simulink model "Offline_DataImport_AND_ECGAnalysis_AND_SCGAnalysis"  (R2020b)
settings: Solver=FixedStepDiscrete  StartTime=0.0  StopTime=param_sim_time  FixedStep=1/fs  MaxStep=1/fs  RelTol=1e-3
undefined symbols (not defined in the file): analyses, fdesignblkfcn, fs, gcbh, param_tot_samples
libraries: dspstat3 x1
(part 1 of 5)
settings Model: PacingRate=100  Creator=rcord  LastModifiedBy=Rafael
settings SolverCC: ZeroCrossControl=DisableAll
settings DataIOCC: ExternalInput=[t, signals.ecg.input, signals.scg.input_x, signals.scg.input_y, signals.scg.input_z]  LoadExternalInput=on  SignalLogging=off  DSMLogging=off  SaveTime=off  ReturnWorkspaceOutputs=off  TimeSaveName=t_preprocessing  OutputSaveName=out_preprocessing  LoggingIntervals=[-inf,inf]
settings SFSimCC: CustomCodeUndefinedFunction=UseInterfaceOnly

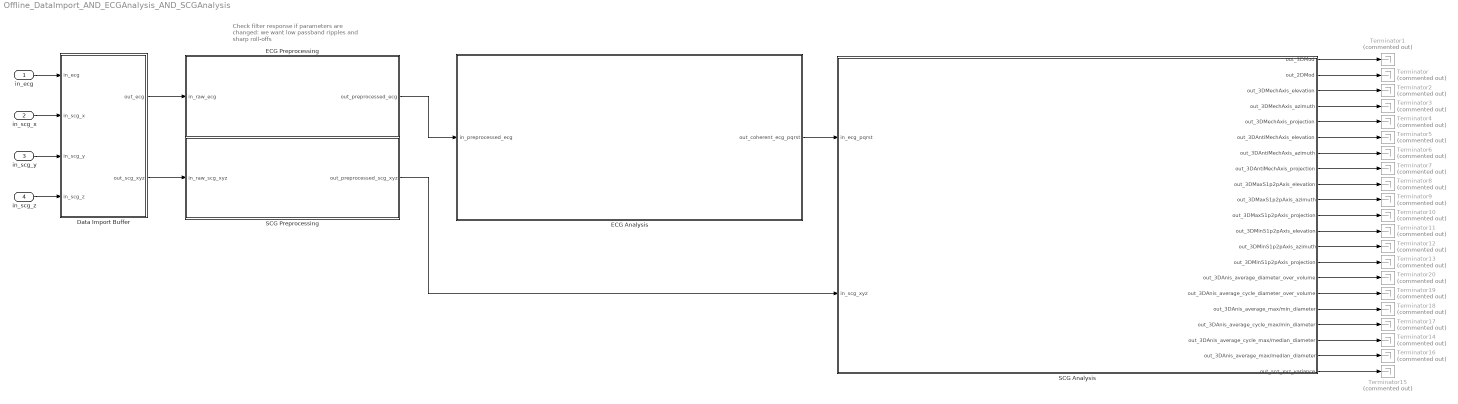
== system Offline_DataImport_AND_ECGAnalysis_AND_SCGAnalysis ==
  note: Check filter response if parameters are changed:
      | we want low passband ripples and sharp roll-offs
  in_ecg : Inport  SampleTime=1/fs
  in_scg_x : Inport  Port=2  SampleTime=1/fs
  in_scg_y : Inport  Port=3  SampleTime=1/fs
  in_scg_z : Inport  Port=4  SampleTime=1/fs
  Data Import Buffer : Subsystem
  ECG Analysis : Subsystem
      mask Display: image('C:\Users\Rafael\Dropbox\Post-Doc Research\ECG Analysis.jpg.png'); % Use "Edit Image" on toolstrip to change.
  ECG Preprocessing : Subsystem  mask{param_ecg_gain_mv=1000, param_ecg_fc_lo=2.05, param_ecg_fc_hi=36, param_ecg_trans_bw=2}
      mask prompts: param_ecg_gain_mv "mV Conversion Gain"; param_ecg_fc_lo "Low Passband Frequency Corner (Hz)"; param_ecg_fc_hi "High Passband Frequency Corner (Hz)"; param_ecg_trans_bw "Transition Bandwidth (Hz)"
      mask init:
      | assignin('base','param_ecg_gain_mv',param_ecg_gain_mv)
      | assignin('base','param_ecg_fc_lo',param_ecg_fc_lo)
      | assignin('base','param_ecg_fc_hi',param_ecg_fc_hi)
      | assignin('base','param_ecg_trans_bw',param_ecg_trans_bw)
      mask DialogControl DescGroupVar Prompt: ECG Preprocessing
      mask DialogControl DescTextVar Prompt: Preprocessing stage of the ECG. This involves conversion from V to mV and a filtfilt operation (i.e. a zero-phase FIR filtering) specified by the passband cornerns and transition bandwidth.
      mask Display: image('PreprocessingSymbol.jpg');
  SCG Analysis : Subsystem
      mask Display: image('C:\Users\Rafael\Dropbox\Post-Doc Research\SCG Analysis.png'); % Use "Edit Image" on toolstrip to change.
  SCG Preprocessing : Subsystem  mask{param_scg_gain_mg=3333, param_scg_fc_lo=7.5, param_scg_fc_hi=40, param_scg_trans_bw=2.5}
      mask prompts: param_scg_gain_mg "V to mg Conversion Gain"; param_scg_fc_lo "Low Passband Frequency Corner (Hz)"; param_scg_fc_hi "High Passband Frequency Corner (Hz)"; param_scg_trans_bw "Transition bandwidth"
      mask init:
      | assignin('base','param_scg_gain_mg',param_scg_gain_mg)
      | assignin('base','param_scg_fc_lo',param_scg_fc_lo)
      | assignin('base','param_scg_fc_hi',param_scg_fc_hi)
      | assignin('base','param_scg_trans_bw',param_scg_trans_bw)
      mask DialogControl DescGroupVar Prompt: SCG Preprocessing
      mask DialogControl DescTextVar Prompt: The SCG (x, y, and z) preprocessing block. This involves a V to mg conversion (determined by the transducer sensitivity) and a filtfilt operation. This filtfilt operation consists of a zero-phase FIR front-back filtering that is identical for each of the three cartesian acceleration components and is specified by the passband frequency corners and the transition bandwidth.
      mask Display: image('PreprocessingSymbol.jpg');
  Terminator{,1..20} (21 alike) : Terminator  Commented=on
  wires:
  in_ecg/1 -> Data Import Buffer/1(in_ecg)
  in_scg_x/1 -> Data Import Buffer/2(in_scg_x)
  in_scg_y/1 -> Data Import Buffer/3(in_scg_y)
  in_scg_z/1 -> Data Import Buffer/4(in_scg_z)
  Data Import Buffer/2(out_scg_xyz) -> SCG Preprocessing/1(in_raw_scg_xyz)
  Data Import Buffer/1(out_ecg) -> ECG Preprocessing/1(in_raw_ecg)
  ECG Preprocessing/1(out_preprocessed_ecg) -> ECG Analysis/1(in_preprocessed_ecg)
  SCG Preprocessing/1(out_preprocessed_scg_xyz) -> SCG Analysis/2(in_scg_xyz)
  ECG Analysis/1(out_coherent_ecg_pqrst) -> SCG Analysis/1(in_ecg_pqrst)
  SCG Analysis/1(out_3DMod) -> Terminator1/1
  SCG Analysis/2(out_2DMod) -> Terminator/1
  SCG Analysis/3(out_3DMechAxis_elevation) -> Terminator2/1
  SCG Analysis/4(out_3DMechAxis_azimuth) -> Terminator3/1
  SCG Analysis/5(out_3DMechAxis_projection) -> Terminator4/1
  SCG Analysis/6(out_3DAntiMechAxis_elevation) -> Terminator5/1
  SCG Analysis/7(out_3DAntiMechAxis_azimuth) -> Terminator6/1
  SCG Analysis/8(out_3DAntiMechAxis_projection) -> Terminator7/1
  SCG Analysis/9(out_3DMaxS1p2pAxis_elevation) -> Terminator8/1
  SCG Analysis/10(out_3DMaxS1p2pAxis_azimuth) -> Terminator9/1
  SCG Analysis/11(out_3DMaxS1p2pAxis_projection) -> Terminator10/1
  SCG Analysis/12(out_3DMinS1p2pAxis_elevation) -> Terminator11/1
  SCG Analysis/13(out_3DMinS1p2pAxis_azimuth) -> Terminator12/1
  SCG Analysis/14(out_3DMinS1p2pAxis_projection) -> Terminator13/1
  SCG Analysis/19(out_3DAnis_average_cycle_max/median_diameter) -> Terminator14/1
  SCG Analysis/21(out_scg_xyz_variance) -> Terminator15/1
  SCG Analysis/20(out_3DAnis_average_max/median_diameter) -> Terminator16/1
  SCG Analysis/18(out_3DAnis_average_cycle_max/min_diameter) -> Terminator17/1
  SCG Analysis/17(out_3DAnis_average_max/min_diameter) -> Terminator18/1
  SCG Analysis/16(out_3DAnis_average_cycle_diameter_over_volume) -> Terminator19/1
  SCG Analysis/15(out_3DAnis_average_diameter_over_volume) -> Terminator20/1

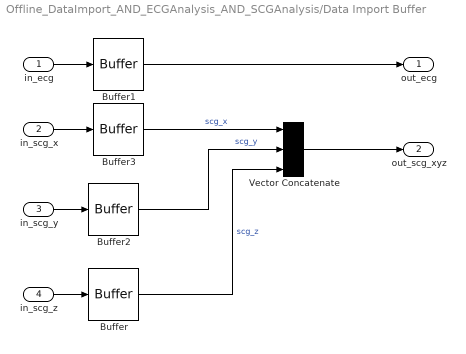
== system Offline_DataImport_AND_ECGAnalysis_AND_SCGAnalysis/Data Import Buffer ==
  in_ecg : Inport
  in_scg_x : Inport  Port=2
  in_scg_y : Inport  Port=3
  in_scg_z : Inport  Port=4
  Buffer{,1..3} (4 alike) : Buffer  N=param_tot_samples  OutputFrames=off
  Vector Concatenate : Concatenate  NumInputs=3  Mode=Multidimensional array  ConcatenateDimension=2
  out_ecg : Outport  VectorParamsAs1DForOutWhenUnconnected=off
  out_scg_xyz : Outport  Port=2  VectorParamsAs1DForOutWhenUnconnected=off
  wires:
  in_ecg/1 -> Buffer1/1
  Buffer/1 -> Vector Concatenate/3  "scg_z"
  Buffer3/1 -> Vector Concatenate/1  "scg_x"
  in_scg_x/1 -> Buffer3/1
  Vector Concatenate/1 -> out_scg_xyz/1
  Buffer1/1 -> out_ecg/1
  Buffer2/1 -> Vector Concatenate/2  "scg_y"
  in_scg_z/1 -> Buffer/1
  in_scg_y/1 -> Buffer2/1

== system Offline_DataImport_AND_ECGAnalysis_AND_SCGAnalysis/ECG Analysis ==
  in_preprocessed_ecg : Inport
  Enabled ECG Analysis Subsystem : Subsystem  TreatAsAtomicUnit=on
  out_coherent_ecg_pqrst : Outport
  wires:
  in_preprocessed_ecg/1 -> Enabled ECG Analysis Subsystem/Enable
  Enabled ECG Analysis Subsystem/1(coherent_ecg_pqrst) -> out_coherent_ecg_pqrst/1

== system Offline_DataImport_AND_ECGAnalysis_AND_SCGAnalysis/ECG Preprocessing ==
  in_raw_ecg : Inport
  Enabled ECG Preprocessing Subsystem : Subsystem  TreatAsAtomicUnit=on
  out_preprocessed_ecg : Outport  VectorParamsAs1DForOutWhenUnconnected=off
  wires:
  Enabled ECG Preprocessing Subsystem/1(Output) -> out_preprocessed_ecg/1
  in_raw_ecg/1 -> Enabled ECG Preprocessing Subsystem/Enable

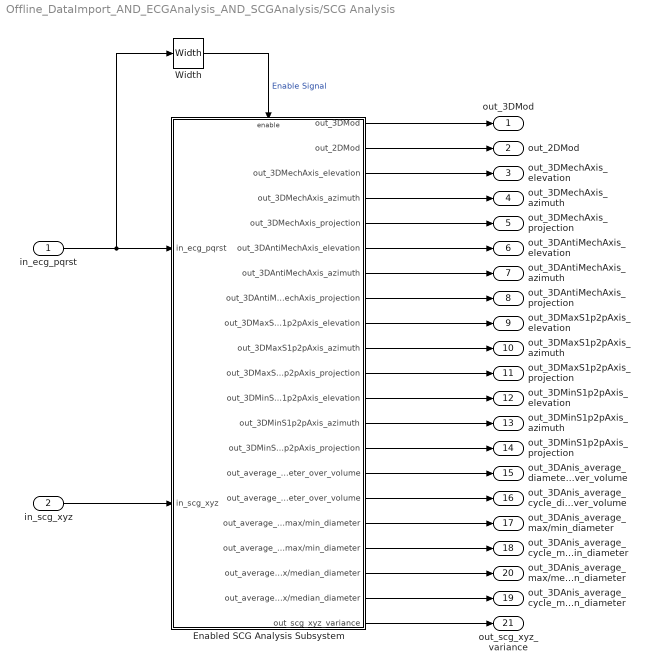
== system Offline_DataImport_AND_ECGAnalysis_AND_SCGAnalysis/SCG Analysis ==
  in_ecg_pqrst : Inport
  in_scg_xyz : Inport  Port=2
  Enabled SCG Analysis Subsystem : Subsystem  TreatAsAtomicUnit=on
  "Width " : Width
  out_3DMod : Outport  VectorParamsAs1DForOutWhenUnconnected=off
  out_2DMod : Outport  Port=2  VectorParamsAs1DForOutWhenUnconnected=off
  out_3DMechAxis_elevation : Outport  Port=3  VectorParamsAs1DForOutWhenUnconnected=off
  out_3DMechAxis_azimuth : Outport  Port=4  VectorParamsAs1DForOutWhenUnconnected=off
  out_3DMechAxis_projection : Outport  Port=5  VectorParamsAs1DForOutWhenUnconnected=off
  out_3DAntiMechAxis_elevation : Outport  Port=6  VectorParamsAs1DForOutWhenUnconnected=off
  out_3DAntiMechAxis_azimuth : Outport  Port=7  VectorParamsAs1DForOutWhenUnconnected=off
  out_3DAntiMechAxis_projection : Outport  Port=8  VectorParamsAs1DForOutWhenUnconnected=off
  out_3DMaxS1p2pAxis_elevation : Outport  Port=9  VectorParamsAs1DForOutWhenUnconnected=off
  out_3DMaxS1p2pAxis_azimuth : Outport  Port=10  VectorParamsAs1DForOutWhenUnconnected=off
  out_3DMaxS1p2pAxis_projection : Outport  Port=11  VectorParamsAs1DForOutWhenUnconnected=off
  out_3DMinS1p2pAxis_elevation : Outport  Port=12  VectorParamsAs1DForOutWhenUnconnected=off
  out_3DMinS1p2pAxis_azimuth : Outport  Port=13  VectorParamsAs1DForOutWhenUnconnected=off
  out_3DMinS1p2pAxis_projection : Outport  Port=14  VectorParamsAs1DForOutWhenUnconnected=off
  out_3DAnis_average_diameter_over_volume : Outport  Port=15  VectorParamsAs1DForOutWhenUnconnected=off
  out_3DAnis_average_cycle_diameter_over_volume : Outport  Port=16  VectorParamsAs1DForOutWhenUnconnected=off
  out_3DAnis_average_max/min_diameter : Outport  Port=17  VectorParamsAs1DForOutWhenUnconnected=off
  out_3DAnis_average_cycle_max/min_diameter : Outport  Port=18  VectorParamsAs1DForOutWhenUnconnected=off
  out_3DAnis_average_cycle_max/median_diameter : Outport  Port=19  VectorParamsAs1DForOutWhenUnconnected=off
  out_3DAnis_average_max/median_diameter : Outport  Port=20  VectorParamsAs1DForOutWhenUnconnected=off
  out_scg_xyz_variance : Outport  Port=21  VectorParamsAs1DForOutWhenUnconnected=off
  wires:
  Enabled SCG Analysis Subsystem/1(out_3DMod) -> out_3DMod/1
  Enabled SCG Analysis Subsystem/2(out_2DMod) -> out_2DMod/1
  in_scg_xyz/1 -> Enabled SCG Analysis Subsystem/2(in_scg_xyz)
  in_ecg_pqrst/1 -> "Width "/1, Enabled SCG Analysis Subsystem/1(in_ecg_pqrst)
  "Width "/1 -> Enabled SCG Analysis Subsystem/Enable  "Enable Signal"
  Enabled SCG Analysis Subsystem/3(out_3DMechAxis_elevation) -> out_3DMechAxis_elevation/1
  Enabled SCG Analysis Subsystem/4(out_3DMechAxis_azimuth) -> out_3DMechAxis_azimuth/1
  Enabled SCG Analysis Subsystem/14(out_3DMinS1p2pAxis_projection) -> out_3DMinS1p2pAxis_projection/1
  Enabled SCG Analysis Subsystem/13(out_3DMinS1p2pAxis_azimuth) -> out_3DMinS1p2pAxis_azimuth/1
  Enabled SCG Analysis Subsystem/12(out_3DMinS1p2pAxis_elevation) -> out_3DMinS1p2pAxis_elevation/1
  Enabled SCG Analysis Subsystem/11(out_3DMaxS1p2pAxis_projection) -> out_3DMaxS1p2pAxis_projection/1
  Enabled SCG Analysis Subsystem/10(out_3DMaxS1p2pAxis_azimuth) -> out_3DMaxS1p2pAxis_azimuth/1
  Enabled SCG Analysis Subsystem/9(out_3DMaxS1p2pAxis_elevation) -> out_3DMaxS1p2pAxis_elevation/1
  Enabled SCG Analysis Subsystem/8(out_3DAntiMechAxis_projection) -> out_3DAntiMechAxis_projection/1
  Enabled SCG Analysis Subsystem/7(out_3DAntiMechAxis_azimuth) -> out_3DAntiMechAxis_azimuth/1
  Enabled SCG Analysis Subsystem/6(out_3DAntiMechAxis_elevation) -> out_3DAntiMechAxis_elevation/1
  Enabled SCG Analysis Subsystem/5(out_3DMechAxis_projection) -> out_3DMechAxis_projection/1
  Enabled SCG Analysis Subsystem/20(out_average_cycle_cycle_max/median_diameter) -> out_3DAnis_average_cycle_max/median_diameter/1
  Enabled SCG Analysis Subsystem/15(out_average_diameter_over_volume) -> out_3DAnis_average_diameter_over_volume/1
  Enabled SCG Analysis Subsystem/21(out_scg_xyz_variance) -> out_scg_xyz_variance/1
  Enabled SCG Analysis Subsystem/16(out_average_cycle_diameter_over_volume) -> out_3DAnis_average_cycle_diameter_over_volume/1
  Enabled SCG Analysis Subsystem/17(out_average_max/min_diameter) -> out_3DAnis_average_max/min_diameter/1
  Enabled SCG Analysis Subsystem/18(out_average_cycle_max/min_diameter) -> out_3DAnis_average_cycle_max/min_diameter/1
  Enabled SCG Analysis Subsystem/19(out_average_max/median_diameter) -> out_3DAnis_average_max/median_diameter/1

== system Offline_DataImport_AND_ECGAnalysis_AND_SCGAnalysis/SCG Preprocessing ==
  in_raw_scg_xyz : Inport
  Enabled SCG Preprocessing Subsystem : Subsystem  TreatAsAtomicUnit=on
  out_preprocessed_scg_xyz : Outport  VectorParamsAs1DForOutWhenUnconnected=off
  wires:
  Enabled SCG Preprocessing Subsystem/1(out_preprocessed_scg_xyz) -> out_preprocessed_scg_xyz/1
  in_raw_scg_xyz/1 -> Enabled SCG Preprocessing Subsystem/Enable

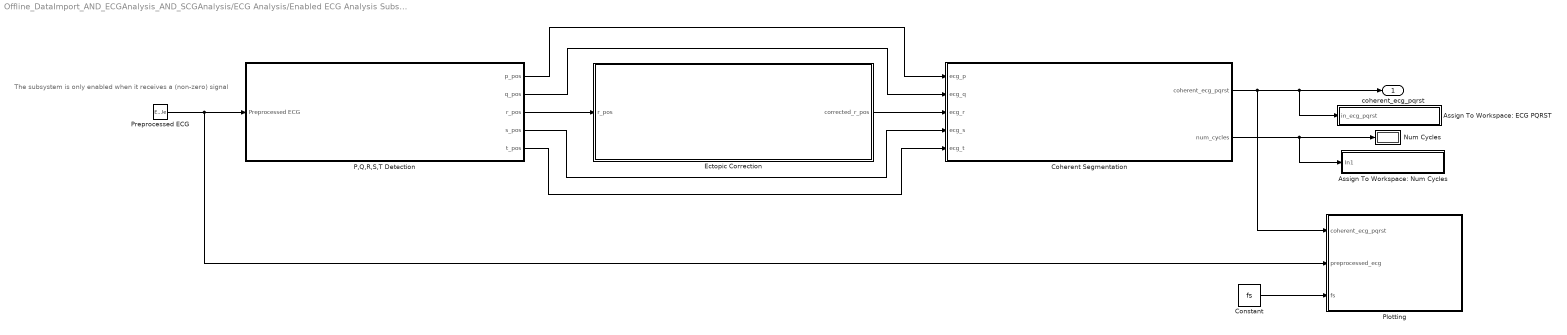
== system Offline_DataImport_AND_ECGAnalysis_AND_SCGAnalysis/ECG Analysis/Enabled ECG Analysis Subsystem ==
  note: The subsystem is only enabled when it receives a (non-zero) signal
  Preprocessed ECG : EnablePort  PropagateVarSize=During execution  ShowOutputPort=on
  Assign To Workspace: ECG PQRST : Subsystem
      mask Display: disp('Assign: out_ecg_pqrst')
  Assign To Workspace: Num Cycles : Subsystem
      mask Display: disp('Assign: out_ecg_num_cycles')
  Coherent Segmentation : Subsystem
      mask Display: image('C:\Users\Rafael\Dropbox\Post-Doc Research\Coherent ECG.jpg'); % Use "Edit Image" on toolstrip to change.
  Constant : Constant  Value=fs
  Ectopic Correction : Subsystem  mask{max_hr=200, max_rr_dev=40}
      mask prompts: max_hr "Maximum Heart Rate (in bpm)"; max_rr_dev "Maximum RR Deviation (in bpm)"
      mask DialogControl DescGroupVar Prompt: Ectopic Correction
      mask DialogControl DescTextVar Prompt: Specify the ectopic detection parameters. What will be defined as an ectopic cycle and removed from further analysis? Maximum heart rate specifies the upper limit of heart rate - any cycles with RR intervals corresponding to heart rates above this limit will be considered ectopic. Maximum RR deviation - any cycles with RR intervals greater or less than this deviation from the average RR will be considered ectopic.
      mask Display: image('C:\Users\Rafael\Dropbox\Post-Doc Research\Tachogram.jpg'); % Use "Edit Image" on toolstrip to change.
  Num Cycles : Display
  P,Q,R,S,T Detection : Subsystem  mask{ecg_algo=PQRST waves - Multi-level Teager Energy Operator}
      mask prompts: ecg_algo "Choose one:"
      mask init:
      | if ecg_algo == 1
      |     param_ecg_algo = 'Pan-Tompkins';
      | elseif ecg_algo == 2
      |     param_ecg_algo = 'Phase Space';
      | elseif ecg_algo == 3
      |     param_ecg_algo = 'Filter Bank';
      | elseif ecg_algo == 4
      |     param_ecg_algo = 'State Machine';
      | elseif ecg_algo == 5
      |     param_ecg_algo = 'Multi-level Teager Energy Operator';
      | end
      | 
      | assignin('base','param_ecg_algo', param_ecg_algo)
      mask TypeOptions ecg_algo: R wave  - Pan-Tompkins | R wave - Phase space | R wave - Filter bank | QRST waves - State machine | PQRST waves - Multi-level Teager Energy Operator
      mask DialogControl DescGroupVar Prompt: ECG PQRST Detection
      mask DialogControl DescTextVar Prompt: Select detected waveform(s) and corresponding detection aglorithm.
      mask DialogControl ParameterGroupVar Prompt: Desired wave(s) and Algorithm
      mask Display: image('C:\Users\Rafael\Dropbox\Post-Doc Research\Labelled ECG.jpg'); % Use "Edit Image" on toolstrip to change.
  Plotting : MATLAB Function  TreatAsAtomicUnit=on
  coherent_ecg_pqrst : Outport
  wires:
  Preprocessed ECG/1 -> P,Q,R,S,T Detection/1(Preprocessed ECG), Plotting/2(preprocessed_ecg)
  P,Q,R,S,T Detection/3(r_pos) -> Ectopic Correction/1(r_pos)
  Constant/1 -> Plotting/3(fs)
  Coherent Segmentation/2(num_cycles) -> Assign To Workspace: Num Cycles/1(In1), Num Cycles/1
  Ectopic Correction/1(corrected_r_pos) -> Coherent Segmentation/3(ecg_r)
  Coherent Segmentation/1(coherent_ecg_pqrst) -> Assign To Workspace: ECG PQRST/1(in_ecg_pqrst), coherent_ecg_pqrst/1, Plotting/1(coherent_ecg_pqrst)
  P,Q,R,S,T Detection/5(t_pos) -> Coherent Segmentation/5(ecg_t)
  P,Q,R,S,T Detection/4(s_pos) -> Coherent Segmentation/4(ecg_s)
  P,Q,R,S,T Detection/1(p_pos) -> Coherent Segmentation/1(ecg_p)
  P,Q,R,S,T Detection/2(q_pos) -> Coherent Segmentation/2(ecg_q)

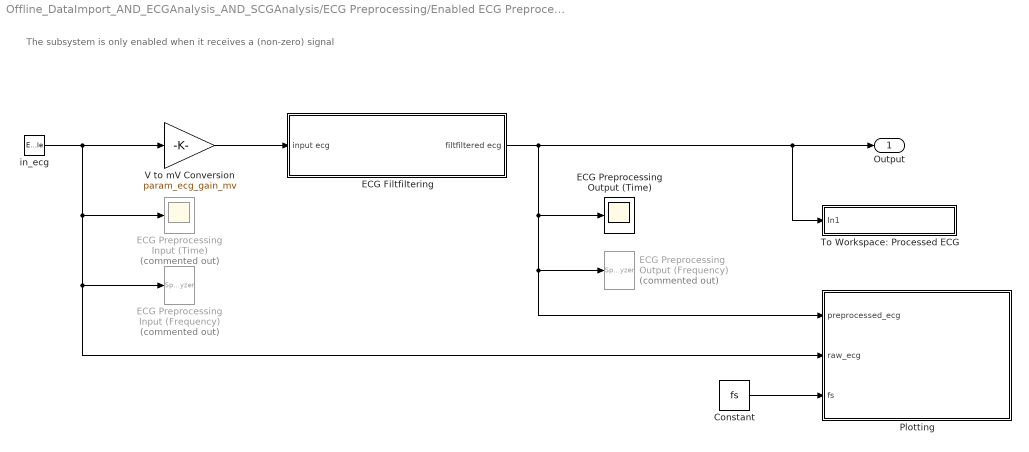
== system Offline_DataImport_AND_ECGAnalysis_AND_SCGAnalysis/ECG Preprocessing/Enabled ECG Preprocessing Subsystem ==
  note: The subsystem is only enabled when it receives a (non-zero) signal
  in_ecg : EnablePort  ShowOutputPort=on
  Constant : Constant  Value=fs
  ECG Filtfiltering : Subsystem
  ECG Preprocessing Input (Frequency) : SpectrumAnalyzer  Commented=on
  ECG Preprocessing Input (Time) : Scope  Commented=on
  ECG Preprocessing Output (Frequency) : SpectrumAnalyzer  Commented=on
  ECG Preprocessing Output (Time) : Scope
  Plotting : MATLAB Function  TreatAsAtomicUnit=on
  To Workspace: Processed ECG : Subsystem
      mask Display: disp('out_ecg_preprocessing')
  V to mV Conversion : Gain  Gain=param_ecg_gain_mv
  Output : Outport  VectorParamsAs1DForOutWhenUnconnected=off
  wires:
  V to mV Conversion/1 -> ECG Filtfiltering/1(input ecg)
  in_ecg/1 -> V to mV Conversion/1, ECG Preprocessing Input (Time)/1, Plotting/2(raw_ecg), ECG Preprocessing Input (Frequency)/1
  ECG Filtfiltering/1(filtfiltered ecg) -> To Workspace: Processed ECG/1(In1), Output/1, ECG Preprocessing Output (Time)/1, Plotting/1(preprocessed_ecg), ECG Preprocessing Output (Frequency)/1
  Constant/1 -> Plotting/3(fs)

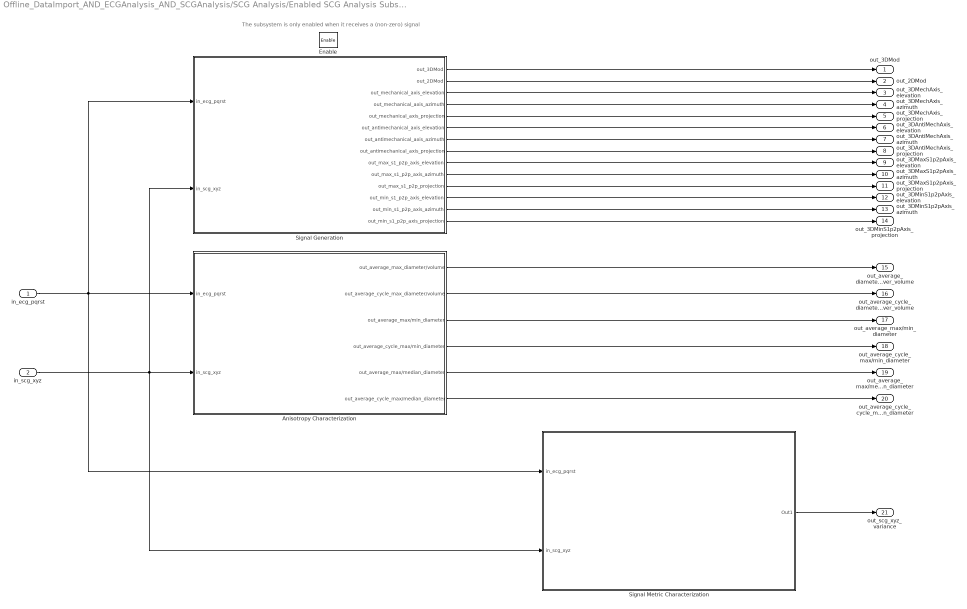
== system Offline_DataImport_AND_ECGAnalysis_AND_SCGAnalysis/SCG Analysis/Enabled SCG Analysis Subsystem ==
  note: The subsystem is only enabled when it receives a (non-zero) signal
  in_ecg_pqrst : Inport
  in_scg_xyz : Inport  Port=2
  Enable : EnablePort  StatesWhenEnabling=reset  PropagateVarSize=During execution
  Anisotropy Characterization : Subsystem
      mask Display: image('C:\Users\Rafael\Dropbox\Post-Doc Research\Anisotropy.png'); % Use "Edit Image" on toolstrip to change.
  Signal Generation : Subsystem
      mask Display: image('C:\Users\Rafael\Dropbox\Post-Doc Research\Signal Generation.png'); % Use "Edit Image" on toolstrip to change.
  Signal Metric Characterization : Subsystem
      mask Display: image('C:\Users\Rafael\Dropbox\Post-Doc Research\SCGAnalysisSymbol.jpg'); % Use "Edit Image" on toolstrip to change.
  out_3DMod : Outport  VectorParamsAs1DForOutWhenUnconnected=off
  out_2DMod : Outport  Port=2  VectorParamsAs1DForOutWhenUnconnected=off
  out_3DMechAxis_elevation : Outport  Port=3  VectorParamsAs1DForOutWhenUnconnected=off
  out_3DMechAxis_azimuth : Outport  Port=4  VectorParamsAs1DForOutWhenUnconnected=off
  out_3DMechAxis_projection : Outport  Port=5  VectorParamsAs1DForOutWhenUnconnected=off
  out_3DAntiMechAxis_elevation : Outport  Port=6  VectorParamsAs1DForOutWhenUnconnected=off
  out_3DAntiMechAxis_azimuth : Outport  Port=7  VectorParamsAs1DForOutWhenUnconnected=off
  out_3DAntiMechAxis_projection : Outport  Port=8  VectorParamsAs1DForOutWhenUnconnected=off
  out_3DMaxS1p2pAxis_elevation : Outport  Port=9  VectorParamsAs1DForOutWhenUnconnected=off
  out_3DMaxS1p2pAxis_azimuth : Outport  Port=10  VectorParamsAs1DForOutWhenUnconnected=off
  out_3DMaxS1p2pAxis_projection : Outport  Port=11  VectorParamsAs1DForOutWhenUnconnected=off
  out_3DMinS1p2pAxis_elevation : Outport  Port=12  VectorParamsAs1DForOutWhenUnconnected=off
  out_3DMinS1p2pAxis_azimuth : Outport  Port=13  VectorParamsAs1DForOutWhenUnconnected=off
  out_3DMinS1p2pAxis_projection : Outport  Port=14  VectorParamsAs1DForOutWhenUnconnected=off
  out_average_diameter_over_volume : Outport  Port=15  VectorParamsAs1DForOutWhenUnconnected=off
  out_average_cycle_diameter_over_volume : Outport  Port=16  VectorParamsAs1DForOutWhenUnconnected=off
  out_average_max/min_diameter : Outport  Port=17  VectorParamsAs1DForOutWhenUnconnected=off
  out_average_cycle_max/min_diameter : Outport  Port=18  VectorParamsAs1DForOutWhenUnconnected=off
  out_average_max/median_diameter : Outport  Port=19  VectorParamsAs1DForOutWhenUnconnected=off
  out_average_cycle_cycle_max/median_diameter : Outport  Port=20  VectorParamsAs1DForOutWhenUnconnected=off
  out_scg_xyz_variance : Outport  Port=21  VectorParamsAs1DForOutWhenUnconnected=off
  wires:
  Signal Generation/2(out_2DMod) -> out_2DMod/1
  Signal Generation/1(out_3DMod) -> out_3DMod/1
  in_scg_xyz/1 -> Signal Generation/2(in_scg_xyz), Signal Metric Characterization/2(in_scg_xyz), Anisotropy Characterization/2(in_scg_xyz)
  in_ecg_pqrst/1 -> Anisotropy Characterization/1(in_ecg_pqrst), Signal Generation/1(in_ecg_pqrst), Signal Metric Characterization/1(in_ecg_pqrst)
  Signal Generation/3(out_mechanical_axis_elevation) -> out_3DMechAxis_elevation/1
  Signal Generation/4(out_mechanical_axis_azimuth) -> out_3DMechAxis_azimuth/1
  Signal Generation/5(out_mechanical_axis_projection) -> out_3DMechAxis_projection/1
  Signal Generation/6(out_antimechanical_axis_elevation) -> out_3DAntiMechAxis_elevation/1
  Signal Generation/7(out_antimechanical_axis_azimuth) -> out_3DAntiMechAxis_azimuth/1
  Signal Generation/8(out_antimechanical_axis_projection) -> out_3DAntiMechAxis_projection/1
  Signal Generation/9(out_max_s1_p2p_axis_elevation) -> out_3DMaxS1p2pAxis_elevation/1
  Signal Generation/10(out_max_s1_p2p_axis_azimuth) -> out_3DMaxS1p2pAxis_azimuth/1
  Signal Generation/11(out_max_s1_p2p_projection) -> out_3DMaxS1p2pAxis_projection/1
  Signal Generation/12(out_min_s1_p2p_axis_elevation) -> out_3DMinS1p2pAxis_elevation/1
  Signal Generation/13(out_min_s1_p2p_axis_azimuth) -> out_3DMinS1p2pAxis_azimuth/1
  Signal Generation/14(out_min_s1_p2p_axis_projection) -> out_3DMinS1p2pAxis_projection/1
  Anisotropy Characterization/1(out_average_max_diameter/volume) -> out_average_diameter_over_volume/1
  Signal Metric Characterization/1(Out1) -> out_scg_xyz_variance/1
  Anisotropy Characterization/2(out_average_cycle_max_diameter/volume) -> out_average_cycle_diameter_over_volume/1
  Anisotropy Characterization/3(out_average_max/min_diameter) -> out_average_max/min_diameter/1
  Anisotropy Characterization/4(out_average_cycle_max/min_diameter) -> out_average_cycle_max/min_diameter/1
  Anisotropy Characterization/5(out_average_max/median_diameter) -> out_average_max/median_diameter/1
  Anisotropy Characterization/6(out_average_cycle_max/median_diameter) -> out_average_cycle_cycle_max/median_diameter/1

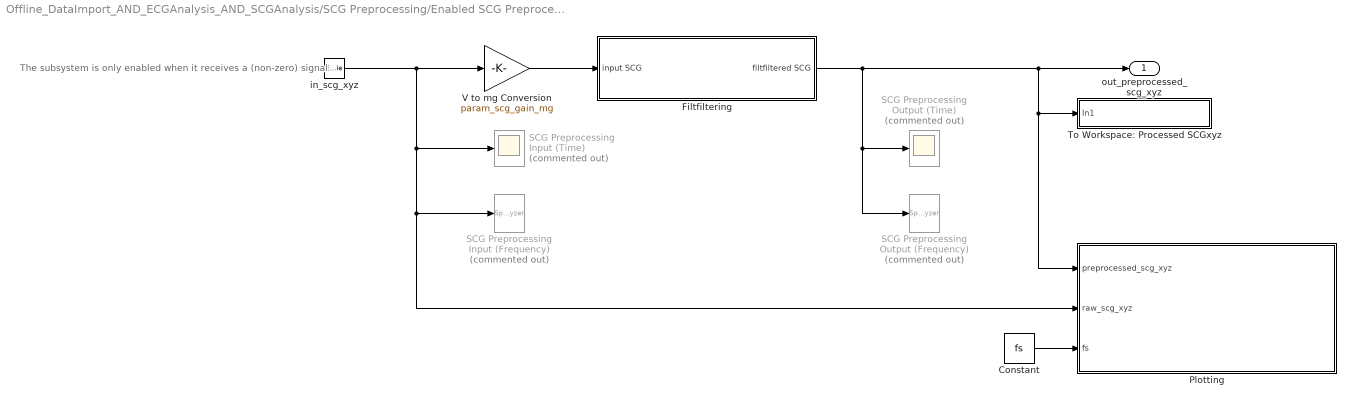
== system Offline_DataImport_AND_ECGAnalysis_AND_SCGAnalysis/SCG Preprocessing/Enabled SCG Preprocessing Subsystem ==
  note: The subsystem is only enabled when it receives a (non-zero) signal
  in_scg_xyz : EnablePort  ShowOutputPort=on
  Constant : Constant  Value=fs
  Filtfiltering : Subsystem
  Plotting : MATLAB Function  TreatAsAtomicUnit=on
  SCG Preprocessing Input (Frequency) : SpectrumAnalyzer  Commented=on
  SCG Preprocessing Input (Time) : Scope  Commented=on
  SCG Preprocessing Output (Frequency) : SpectrumAnalyzer  Commented=on
  SCG Preprocessing Output (Time) : Scope  Commented=on
  To Workspace: Processed SCGxyz : Subsystem
      mask Display: disp('out_scg_xyz_preprocessing')
  V to mg Conversion : Gain  Gain=param_scg_gain_mg
  out_preprocessed_scg_xyz : Outport  VectorParamsAs1DForOutWhenUnconnected=off
  wires:
  V to mg Conversion/1 -> Filtfiltering/1(" input SCG")
  Filtfiltering/1(filtfiltered SCG) -> out_preprocessed_scg_xyz/1, To Workspace: Processed SCGxyz/1(In1), Plotting/1(preprocessed_scg_xyz), SCG Preprocessing Output (Frequency)/1, SCG Preprocessing Output (Time)/1
  Constant/1 -> Plotting/3(fs)
  in_scg_xyz/1 -> V to mg Conversion/1, Plotting/2(raw_scg_xyz), SCG Preprocessing Input (Frequency)/1, SCG Preprocessing Input (Time)/1

== system Offline_DataImport_AND_ECGAnalysis_AND_SCGAnalysis/ECG Analysis/Enabled ECG Analysis Subsystem/Assign To Workspace: ECG PQRST ==
  in_ecg_pqrst : Inport
  Enable Selector : Selector  NumberOfDimensions=2  InputPortWidth=3  IndexOptions=Index vector (dialog),Index vector (dialog)  Indices=[1],[3]  OutputSizes=1,1
  Enabled To Workspace ECG PQRST : Subsystem  TreatAsAtomicUnit=on
  wires:
  in_ecg_pqrst/1 -> Enable Selector/1, Enabled To Workspace ECG PQRST/1(in_ecg_pqrst)
  Enable Selector/1 -> Enabled To Workspace ECG PQRST/Enable  "Enable"

== system Offline_DataImport_AND_ECGAnalysis_AND_SCGAnalysis/ECG Analysis/Enabled ECG Analysis Subsystem/Assign To Workspace: Num Cycles ==
  In1 : Inport
  Enabled To Workspace ECG Num Cycles : Subsystem  TreatAsAtomicUnit=on
  wires:
  In1/1 -> Enabled To Workspace ECG Num Cycles/Enable

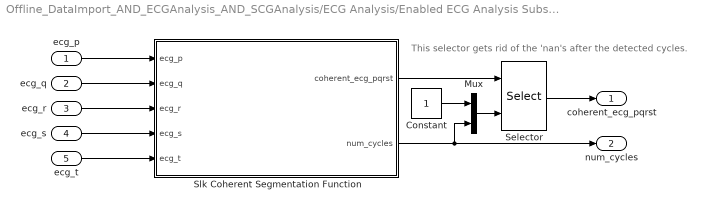
== system Offline_DataImport_AND_ECGAnalysis_AND_SCGAnalysis/ECG Analysis/Enabled ECG Analysis Subsystem/Coherent Segmentation ==
  note: This selector gets rid of the 'nan's after the detected cycles.
  ecg_p : Inport
  ecg_q : Inport  Port=2
  ecg_r : Inport  Port=3
  ecg_s : Inport  Port=4
  ecg_t : Inport  Port=5
  Constant : Constant
  Mux : Mux  Inputs=2
  Selector : Selector  NumberOfDimensions=2  InputPortWidth=3  IndexOptions=Starting and ending indices (port),Index vector (dialog)  Indices=[1 3],[1 2 3 3 5]  OutputSizes=1,1
  Slk Coherent Segmentation Function : MATLAB Function  TreatAsAtomicUnit=on
  coherent_ecg_pqrst : Outport
  num_cycles : Outport  Port=2
  wires:
  ecg_q/1 -> Slk Coherent Segmentation Function/2(ecg_q)
  ecg_s/1 -> Slk Coherent Segmentation Function/4(ecg_s)
  ecg_p/1 -> Slk Coherent Segmentation Function/1(ecg_p)
  ecg_r/1 -> Slk Coherent Segmentation Function/3(ecg_r)
  ecg_t/1 -> Slk Coherent Segmentation Function/5(ecg_t)
  Constant/1 -> Mux/1
  Mux/1 -> Selector/2
  Slk Coherent Segmentation Function/1(coherent_ecg_pqrst) -> Selector/1
  Selector/1 -> coherent_ecg_pqrst/1
  Slk Coherent Segmentation Function/2(num_cycles) -> num_cycles/1, Mux/2

== system Offline_DataImport_AND_ECGAnalysis_AND_SCGAnalysis/ECG Analysis/Enabled ECG Analysis Subsystem/Ectopic Correction ==
  r_pos : Inport
  Constant : Constant  Value=max_hr
  Constant1 : Constant  Value=max_rr_dev
  Constant2 : Constant  Value=fs
  Ectopic Correction : MATLAB Function  TreatAsAtomicUnit=on
  corrected_r_pos : Outport
  wires:
  Ectopic Correction/1(corrected_r_pos) -> corrected_r_pos/1
  Constant2/1 -> Ectopic Correction/1(fs)
  Constant/1 -> Ectopic Correction/2(max_hr)
  Constant1/1 -> Ectopic Correction/3(max_rr_dev)
  r_pos/1 -> Ectopic Correction/4(r_pos)

== system Offline_DataImport_AND_ECGAnalysis_AND_SCGAnalysis/ECG Analysis/Enabled ECG Analysis Subsystem/P,Q,R,S,T Detection ==
  Preprocessed ECG : Inport
  Constant : Constant  Value=fs
  Constant1 : Constant  Value=ecg_algo
  Wrapped BioSigKit ECG PQRST Detection : MATLAB Function  TreatAsAtomicUnit=on
  p_pos : Outport
      settings: VarSizeSig=Yes
  q_pos : Outport  Port=2
      settings: VarSizeSig=Yes
  r_pos : Outport  Port=3
      settings: VarSizeSig=Yes
  s_pos : Outport  Port=4
      settings: VarSizeSig=Yes
  t_pos : Outport  Port=5
      settings: VarSizeSig=Yes
  wires:
  Preprocessed ECG/1 -> Wrapped BioSigKit ECG PQRST Detection/2(preprocessed_ecg)
  Constant/1 -> Wrapped BioSigKit ECG PQRST Detection/1(fs)
  Wrapped BioSigKit ECG PQRST Detection/1(ecg_p) -> p_pos/1
  Wrapped BioSigKit ECG PQRST Detection/2(ecg_q) -> q_pos/1
  Wrapped BioSigKit ECG PQRST Detection/3(ecg_r) -> r_pos/1
  Wrapped BioSigKit ECG PQRST Detection/4(ecg_s) -> s_pos/1
  Wrapped BioSigKit ECG PQRST Detection/5(ecg_t) -> t_pos/1
  Constant1/1 -> Wrapped BioSigKit ECG PQRST Detection/3(ecg_algo)

== system Offline_DataImport_AND_ECGAnalysis_AND_SCGAnalysis/ECG Preprocessing/Enabled ECG Preprocessing Subsystem/ECG Filtfiltering ==
  input ecg : Inport
  Bandpass Filter 1 : Subsystem  DialogController=fdesignblkfcn  InitFcn=fdesignblkfcn(gcbh, {'InitFcn'});  mask(Bandpass Filter){}
      mask help: Design a bandpass filter
      settings: CopyFcn=fdesignblkfcn(gcbh, {'CopyFcn'});
      mask Help: helpview(mapfilelocation('dsp'), 'dspbandpassfilter');
      mask Display: disp('Bandpass');
  Bandpass Filter 2 : Subsystem  DialogController=fdesignblkfcn  InitFcn=fdesignblkfcn(gcbh, {'InitFcn'});  mask(Bandpass Filter){}
      mask help: Design a bandpass filter
      settings: CopyFcn=fdesignblkfcn(gcbh, {'CopyFcn'});
      mask Help: helpview(mapfilelocation('dsp'), 'dspbandpassfilter');
      mask Display: disp('Bandpass');
  Flip : DSPFlip
  Flip1 : DSPFlip
  filtfiltered ecg : Outport  VectorParamsAs1DForOutWhenUnconnected=off
  wires:
  Flip/1 -> Bandpass Filter 2/1(In)
  input ecg/1 -> Bandpass Filter 1/1(In)
  Flip1/1 -> filtfiltered ecg/1
  Bandpass Filter 1/1(Out) -> Flip/1
  Bandpass Filter 2/1(Out) -> Flip1/1

== system Offline_DataImport_AND_ECGAnalysis_AND_SCGAnalysis/ECG Preprocessing/Enabled ECG Preprocessing Subsystem/To Workspace: Processed ECG ==
  In1 : Inport
  Enabled To Workspace ECG Subsystem : Subsystem  TreatAsAtomicUnit=on
  wires:
  In1/1 -> Enabled To Workspace ECG Subsystem/Enable, Enabled To Workspace ECG Subsystem/1(In1)

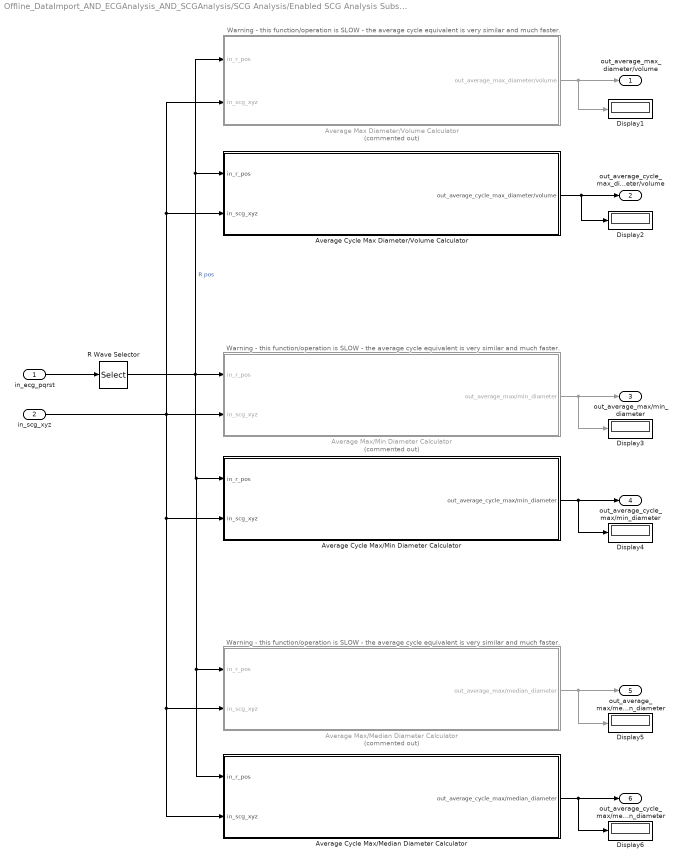
== system Offline_DataImport_AND_ECGAnalysis_AND_SCGAnalysis/SCG Analysis/Enabled SCG Analysis Subsystem/Anisotropy Characterization ==
  note: Warning - this function/operation is SLOW - the average cycle equivalent is very similar and much faster.
  note: Warning - this function/operation is SLOW - the average cycle equivalent is very similar and much faster.
  note: Warning - this function/operation is SLOW - the average cycle equivalent is very similar and much faster.
  in_ecg_pqrst : Inport
  in_scg_xyz : Inport  Port=2
  Average Cycle Max Diameter/Volume Calculator : Subsystem
  Average Cycle Max/Median Diameter Calculator : Subsystem
  Average Cycle Max/Min Diameter Calculator : Subsystem
  Average Max Diameter/Volume Calculator : Subsystem  Commented=on
  Average Max/Median Diameter Calculator : Subsystem  Commented=on
  Average Max/Min Diameter Calculator : Subsystem  Commented=on
  Display{1..6} (6 alike) : Display
  R Wave Selector : Selector  NumberOfDimensions=2  InputPortWidth=3  IndexOptions=Select all,Index vector (dialog)  Indices=[1 3],3  OutputSizes=1,1
  out_average_max_diameter/volume : Outport
  out_average_cycle_max_diameter/volume : Outport  Port=2
  out_average_max/min_diameter : Outport  Port=3
  out_average_cycle_max/min_diameter : Outport  Port=4
  out_average_max/median_diameter : Outport  Port=5
  out_average_cycle_max/median_diameter : Outport  Port=6
  wires:
  Average Max Diameter/Volume Calculator/1(out_average_max_diameter/volume) -> out_average_max_diameter/volume/1, Display1/1
  in_ecg_pqrst/1 -> R Wave Selector/1
  in_scg_xyz/1 -> Average Max Diameter/Volume Calculator/2(in_scg_xyz), Average Cycle Max Diameter/Volume Calculator/2(in_scg_xyz), Average Cycle Max/Median Diameter Calculator/2(in_scg_xyz), Average Max/Median Diameter Calculator/2(in_scg_xyz), Average Cycle Max/Min Diameter Calculator/2(in_scg_xyz), Average Max/Min Diameter Calculator/2(in_scg_xyz)
  Average Cycle Max Diameter/Volume Calculator/1(out_average_cycle_max_diameter/volume) -> Display2/1, out_average_cycle_max_diameter/volume/1
  R Wave Selector/1 -> Average Cycle Max Diameter/Volume Calculator/1(in_r_pos), Average Max Diameter/Volume Calculator/1(in_r_pos), Average Max/Min Diameter Calculator/1(in_r_pos), Average Cycle Max/Median Diameter Calculator/1(in_r_pos), Average Max/Median Diameter Calculator/1(in_r_pos), Average Cycle Max/Min Diameter Calculator/1(in_r_pos)  "R pos"
  Average Max/Min Diameter Calculator/1(out_average_max/min_diameter) -> out_average_max/min_diameter/1, Display3/1
  Average Cycle Max/Min Diameter Calculator/1(out_average_cycle_max/min_diameter) -> Display4/1, out_average_cycle_max/min_diameter/1
  Average Max/Median Diameter Calculator/1(out_average_max/median_diameter) -> Display5/1, out_average_max/median_diameter/1
  Average Cycle Max/Median Diameter Calculator/1(out_average_cycle_max/median_diameter) -> out_average_cycle_max/median_diameter/1, Display6/1

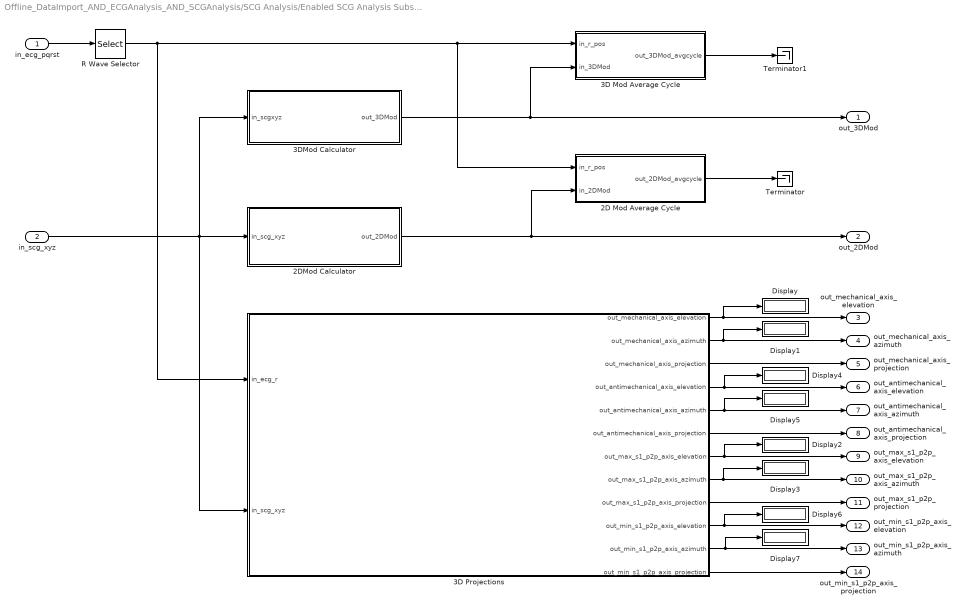
== system Offline_DataImport_AND_ECGAnalysis_AND_SCGAnalysis/SCG Analysis/Enabled SCG Analysis Subsystem/Signal Generation ==
  in_ecg_pqrst : Inport
  in_scg_xyz : Inport  Port=2
  2D Mod Average Cycle : Subsystem
  2DMod Calculator : Subsystem  mask{xyz2Dcombo=xz (transverse plane)}
      mask prompts: xyz2Dcombo "2D component combination:"
      mask init:
      | if xyz2Dcombo == 1
      |     param_2Dxyzcombo = 'xy';
      | elseif xyz2Dcombo == 2
      |     param_2Dxyzcombo = 'yz';
      | elseif xyz2Dcombo == 3
      |     param_2Dxyzcombo = 'xz';
      | end
      | 
      | assignin('base','param_2Dxyzcombo', param_2Dxyzcombo)
      mask TypeOptions xyz2Dcombo: xy (coronal plane) | yz (sagittal plane) | xz (transverse plane)
      mask DialogControl DescGroupVar Prompt: 2D Modulus Calculator
      mask DialogControl DescTextVar Prompt: Subsystem to calculate a 2D modulus signal from a user-specified combination of any two of the SCG x, y, or z components.
  3D Mod Average Cycle : Subsystem
  3D Projections : Subsystem
      mask Display: image('C:\Users\Rafael\Dropbox\Post-Doc Research\Coordinate Frames with Signals.png'); % Use "Edit Image" on toolstrip to change.
  3DMod Calculator : Subsystem
  Display{,1..7} (8 alike) : Display
  R Wave Selector : Selector  NumberOfDimensions=2  InputPortWidth=3  IndexOptions=Select all,Index vector (dialog)  Indices=[1 3],3  OutputSizes=1,1
  Terminator : Terminator
  Terminator1 : Terminator
  out_3DMod : Outport
  out_2DMod : Outport  Port=2
  out_mechanical_axis_elevation : Outport  Port=3
  out_mechanical_axis_azimuth : Outport  Port=4
  out_mechanical_axis_projection : Outport  Port=5
  out_antimechanical_axis_elevation : Outport  Port=6
  out_antimechanical_axis_azimuth : Outport  Port=7
  out_antimechanical_axis_projection : Outport  Port=8
  out_max_s1_p2p_axis_elevation : Outport  Port=9
  out_max_s1_p2p_axis_azimuth : Outport  Port=10
  out_max_s1_p2p_projection : Outport  Port=11
  out_min_s1_p2p_axis_elevation : Outport  Port=12
  out_min_s1_p2p_axis_azimuth : Outport  Port=13
  out_min_s1_p2p_axis_projection : Outport  Port=14
  wires:
  3DMod Calculator/1(out_3DMod) -> out_3DMod/1, 3D Mod Average Cycle/2(in_3DMod)
  2DMod Calculator/1(out_2DMod) -> 2D Mod Average Cycle/2(in_2DMod), out_2DMod/1
  2D Mod Average Cycle/1(out_2DMod_avgcycle) -> Terminator/1
  3D Mod Average Cycle/1(out_3DMod_avgcycle) -> Terminator1/1
  R Wave Selector/1 -> 3D Mod Average Cycle/1(in_r_pos), 2D Mod Average Cycle/1(in_r_pos), 3D Projections/1(in_ecg_r)
  in_ecg_pqrst/1 -> R Wave Selector/1
  in_scg_xyz/1 -> 3DMod Calculator/1(in_scgxyz), 2DMod Calculator/1(in_scg_xyz), 3D Projections/2(in_scg_xyz)
  3D Projections/4(out_antimechanical_axis_elevation) -> out_antimechanical_axis_elevation/1, Display4/1
  3D Projections/2(out_mechanical_axis_azimuth) -> Display1/1, out_mechanical_axis_azimuth/1
  3D Projections/10(out_min_s1_p2p_axis_elevation) -> Display6/1, out_min_s1_p2p_axis_elevation/1
  3D Projections/5(out_antimechanical_axis_azimuth) -> out_antimechanical_axis_azimuth/1, Display5/1
  3D Projections/8(out_max_s1_p2p_axis_azimuth) -> Display3/1, out_max_s1_p2p_axis_azimuth/1
  3D Projections/6(out_antimechanical_axis_projection) -> out_antimechanical_axis_projection/1
  3D Projections/7(out_max_s1_p2p_axis_elevation) -> out_max_s1_p2p_axis_elevation/1, Display2/1
  3D Projections/11(out_min_s1_p2p_axis_azimuth) -> out_min_s1_p2p_axis_azimuth/1, Display7/1
  3D Projections/12(out_min_s1_p2p_axis_projection) -> out_min_s1_p2p_axis_projection/1
  3D Projections/9(out_max_s1_p2p_axis_projection) -> out_max_s1_p2p_projection/1
  3D Projections/1(out_mechanical_axis_elevation) -> Display/1, out_mechanical_axis_elevation/1
  3D Projections/3(out_mechanical_axis_projection) -> out_mechanical_axis_projection/1

== system Offline_DataImport_AND_ECGAnalysis_AND_SCGAnalysis/SCG Analysis/Enabled SCG Analysis Subsystem/Signal Metric Characterization ==
  in_ecg_pqrst : Inport
  in_scg_xyz : Inport  Port=2
  SCG xyz Variance : Display
  Variance : dspstat3/Variance  run=off  InputProcessing=Columns as channels (frame based)  reset_popup=None  directionMode=Each column  dimension=1  roiEnable=off  roiType=Rectangles  roiPortion=Entire ROI  roiOutput=Individual statistics for each ROI  roiFlag=off  roundingMode=Floor  overflowMode=off
  Out1 : Outport
  wires:
  Variance/1 -> Out1/1, SCG xyz Variance/1
  in_scg_xyz/1 -> Variance/1

== system Offline_DataImport_AND_ECGAnalysis_AND_SCGAnalysis/SCG Preprocessing/Enabled SCG Preprocessing Subsystem/Filtfiltering ==
  " input SCG" : Inport
  Bandpass Filter 1 : Subsystem  DialogController=fdesignblkfcn  InitFcn=fdesignblkfcn(gcbh, {'InitFcn'});  mask(Bandpass Filter){}
      mask help: Design a bandpass filter
      settings: CopyFcn=fdesignblkfcn(gcbh, {'CopyFcn'});
      mask Help: helpview(mapfilelocation('dsp'), 'dspbandpassfilter');
      mask Display: disp('Bandpass');
  Bandpass Filter 2 : Subsystem  DialogController=fdesignblkfcn  InitFcn=fdesignblkfcn(gcbh, {'InitFcn'});  mask(Bandpass Filter){}
      mask help: Design a bandpass filter
      settings: CopyFcn=fdesignblkfcn(gcbh, {'CopyFcn'});
      mask Help: helpview(mapfilelocation('dsp'), 'dspbandpassfilter');
      mask Display: disp('Bandpass');
  Flip : DSPFlip
  Flip1 : DSPFlip
  filtfiltered SCG : Outport  VectorParamsAs1DForOutWhenUnconnected=off
  wires:
  Bandpass Filter 2/1(Out) -> Flip1/1
  Bandpass Filter 1/1(Out) -> Flip/1
  Flip1/1 -> filtfiltered SCG/1
  " input SCG"/1 -> Bandpass Filter 1/1(In)
  Flip/1 -> Bandpass Filter 2/1(In)

== system Offline_DataImport_AND_ECGAnalysis_AND_SCGAnalysis/SCG Preprocessing/Enabled SCG Preprocessing Subsystem/To Workspace: Processed SCGxyz ==
  In1 : Inport
  To Workspace SCG Enabled Subsystem : Subsystem  TreatAsAtomicUnit=on
  wires:
  In1/1 -> To Workspace SCG Enabled Subsystem/Enable, To Workspace SCG Enabled Subsystem/1(In1)

== system Offline_DataImport_AND_ECGAnalysis_AND_SCGAnalysis/ECG Analysis/Enabled ECG Analysis Subsystem/Assign To Workspace: ECG PQRST/Enabled To Workspace ECG PQRST ==
  note: Make sure the funtion expects input dimensions of appropriate size.
  note: The subsystem is only enabled when it receives a (non-zero) signal
  in_ecg_pqrst : Inport
  Enable : EnablePort
  Slk Wrapped Assigned to Workspace : MATLAB Function  TreatAsAtomicUnit=on
  wires:
  in_ecg_pqrst/1 -> Slk Wrapped Assigned to Workspace/1(ecg_pqrst)

== system Offline_DataImport_AND_ECGAnalysis_AND_SCGAnalysis/ECG Analysis/Enabled ECG Analysis Subsystem/Assign To Workspace: Num Cycles/Enabled To Workspace ECG Num Cycles ==
  note: Make sure the funtion expects input dimensions of appropriate size.
  note: The subsystem is only enabled when it receives a (non-zero) signal
  Enable : EnablePort  ShowOutputPort=on
  Slk Wrapped Assigned To Workspace : MATLAB Function  TreatAsAtomicUnit=on
  wires:
  Enable/1 -> Slk Wrapped Assigned To Workspace/1(assigned_var)
